simulink model "L0605"  (Simulink 10.2)
settings: Solver=ode45  StartTime=0.0  StopTime=50  MaxStep=0.1  RelTol=1e-3
libraries: simulink x3
settings Model: Creator=Ranci  LastModifiedBy=Ranci
settings DataIOCC: SaveFormat=Dataset  SignalLoggingSaveFormat=Dataset  ReturnWorkspaceOutputs=on
settings OptimizationCC: LifeSpan=auto
settings DebuggingCC: UnderspecifiedInitializationDetection=Simplified  MergeDetectMultiDrivingBlocksExec=error  FcnCallInpInsideContextMsg=error  SFUnexpectedBacktrackingDiag=error  SFNoUnconditionalDefaultTransitionDiag=error  SFExecutionAtInitializationDiag=warning  ArithmeticOperatorsInVariantConditions=error
settings HardwareCC: ProdBitPerPointer=64  ProdBitPerSizeT=64  ProdBitPerPtrDiffT=64  ProdLargestAtomicFloat=Float  ProdIntDivRoundTo=Zero  ProdEndianess=LittleEndian  ProdWordSize=64  ProdHWDeviceType=Intel->x86-64 (Windows64)
settings ModelReferenceCC: PropagateSignalLabelsOutOfModel=on
settings SFSimCC: SimUseLocalCustomCode=on  CustomCodeUndefinedFunction=FilterOut
settings RTWCC: RTWUseLocalCustomCode=on
settings CodeAppCC: StateflowObjectComments=off
settings GRTTargetCC: TargetLangStandard=C99 (ISO)  CombineOutputUpdateFcns=on  GRTInterface=off
settings ConfigComp: CovMetricSettings=dwe  CovSaveCumulativeToWorkspaceVar=off  CovSaveSingleToWorkspaceVar=off  CovExternalEMLEnable=on

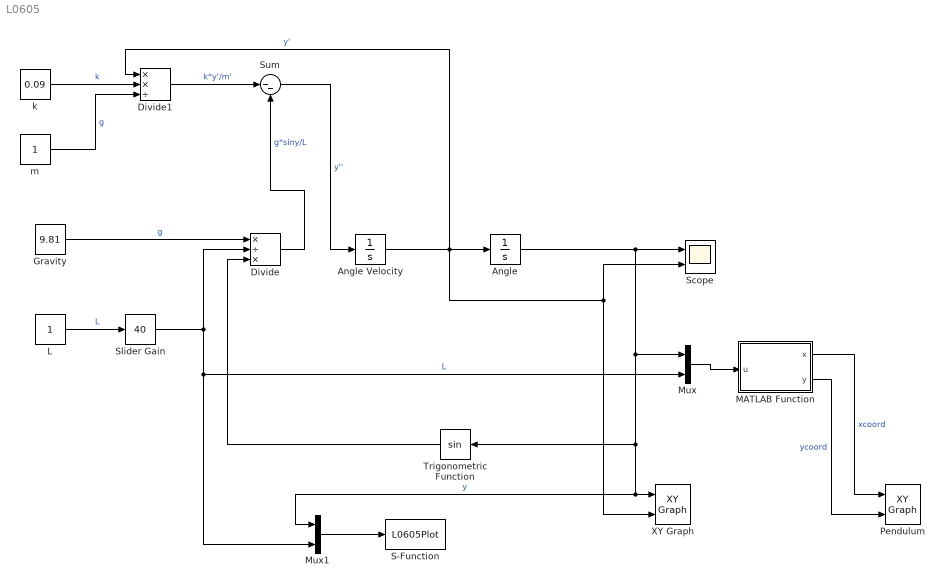
== system L0605 ==
  Angle : Integrator
  Angle Velocity : Integrator  InitialCondition=2
  Divide : Product  Inputs=*/*
  Divide1 : Product  Inputs=**/
  Gravity : Constant  Value=9.81
  L : Constant
  MATLAB Function : MATLAB Function  TreatAsAtomicUnit=on
  Mux : Mux  Inputs=2
  Mux1 : Mux  Inputs=2
  Pendulum : simulink/Sinks/XY Graph  xmin=-15  xmax=15  ymin=-15  ymax=15  st=-1
  S-Function : S-Function  FunctionName=L0605Plot  Parameters=0.1  SFunctionDeploymentMode=off  EnableBusSupport=off
  Scope : Scope  NumInputPorts=2
  Slider Gain : simulink/Math Operations/Slider Gain  gain=40  low=0  high=40
  Sum : Sum  Inputs=|--
  Trigonometric Function : Trigonometry
  XY Graph : simulink/Sinks/XY Graph  xmin=-2  xmax=2  ymin=-2  ymax=2  st=-1
  k : Constant  Value=0.09
  m : Constant
  wires:
  L/1 -> Slider Gain/1  "L"
  Gravity/1 -> Divide/1  "g"
  Slider Gain/1 -> Divide/2, Mux1/2, Mux/2  "L"
  Angle Velocity/1 -> Divide1/1, XY Graph/2, Scope/2, Angle/1  "y'"
  Angle/1 -> Mux/1, Mux1/1, XY Graph/1, Trigonometric Function/1, Scope/1  "y"
  Mux/1 -> MATLAB Function/1(u)
  MATLAB Function/1(x) -> Pendulum/1  "xcoord"
  MATLAB Function/2(y) -> Pendulum/2  "ycoord"
  k/1 -> Divide1/2  "k"
  m/1 -> Divide1/3  "g"
  Divide1/1 -> Sum/1  "k*y'/m'"
  Divide/1 -> Sum/2  "g*siny/L"
  Sum/1 -> Angle Velocity/1  "y''"
  Trigonometric Function/1 -> Divide/3
  Mux1/1 -> S-Function/1

== matlab function MATLAB Function ==
  data: x output double; u input double; y output double
function [x, y] = fcn(u)
x = u(2) * sin(u(1));      %координата х
y = -u(2) * cos(u(1));     %координата y
